simulink model "feedforward_obtencion_datos"  (R2016a)
settings: Solver=VariableStepAuto  StartTime=0.0  StopTime=20  RelTol=1e-3
libraries: simulink x1
settings Model: Creator=Daniel  LastModifiedBy=Daniel

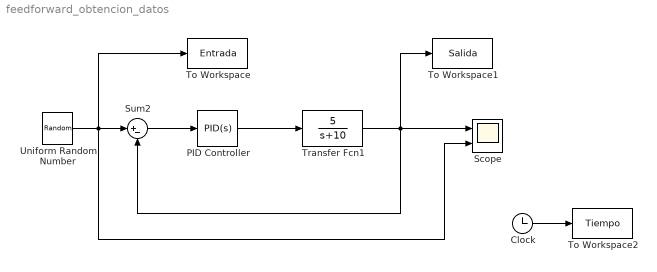
== system feedforward_obtencion_datos ==
  Clock : Clock
  PID Controller : simulink/Continuous/PID Controller  Controller=PID  TimeDomain=Continuous-time  SampleTime=-1  IntegratorMethod=Forward Euler  FilterMethod=Forward Euler  Form=Parallel  UseFilter=on  ControllerParametersSource=internal  P=12.33  I=10  D=0  N=100  InitialConditionSource=internal  InitialConditionForIntegrator=0  InitialConditionForFilter=0  ExternalReset=none  LimitOutput=off  UpperSaturationLimit=inf  LowerSaturationLimit=-inf  LinearizeAsGain=on  AntiWindupMode=none  Kb=1  TrackingMode=off  Kt=1  PParamMin=[]  PParamMax=[]  IParamMin=[]  IParamMax=[]  DParamMin=[]  DParamMax=[]  NParamMin=[]  NParamMax=[]  KbParamMin=[]  KbParamMax=[]  KtParamMin=[]  KtParamMax=[]  POutMin=[]  POutMax=[]  IOutMin=[]  IOutMax=[]  DOutMin=[]  DOutMax=[]  NOutMin=[]  NOutMax=[]  KbOutMin=[]  KbOutMax=[]  KtOutMin=[]  KtOutMax=[]  IntegratorOutMin=[]  IntegratorOutMax=[]  FilterOutMin=[]  FilterOutMax=[]  SumOutMin=[]  SumOutMax=[]  SumI1OutMin=[]  SumI1OutMax=[]  SumI2OutMin=[]  SumI2OutMax=[]  SumI3OutMin=[]  SumI3OutMax=[]  SumDOutMin=[]  SumDOutMax=[]  SaturationOutMin=[]  SaturationOutMax=[]  IntegratorContinuousStateAttributes=''  IntegratorStateMustResolveToSignalObject=off  IntegratorRTWStateStorageClass=Auto  FilterContinuousStateAttributes=''  FilterStateMustResolveToSignalObject=off  FilterRTWStateStorageClass=Auto  DifferentiatorICPrevScaledInput=0  DifferentiatorOutMin=[]  DifferentiatorOutMax=[]
  Scope : Scope  NumInputPorts=2
  Sum2 : Sum  Inputs=|+-
  To Workspace : ToWorkspace  VariableName=Entrada  SampleTime=0.01
  To Workspace1 : ToWorkspace  VariableName=Salida  SampleTime=0.01
  To Workspace2 : ToWorkspace  VariableName=Tiempo  SampleTime=0.01
  Transfer Fcn1 : TransferFcn  Numerator=[5]  Denominator=[1 10]
  Uniform Random Number : UniformRandomNumber  Minimum=0  Maximum=5  SampleTime=0.5
  wires:
  Sum2/1 -> PID Controller/1
  PID Controller/1 -> Transfer Fcn1/1
  Uniform Random Number/1 -> Scope/2, To Workspace/1, Sum2/1
  Transfer Fcn1/1 -> To Workspace1/1, Scope/1, Sum2/2
  Clock/1 -> To Workspace2/1
